simulink model "Hw1_4"  (R2015b)
settings: Solver=VariableStepAuto  StartTime=0.0  StopTime=5000  RelTol=1e-3
settings Model: Creator=user  LastModifiedBy=user

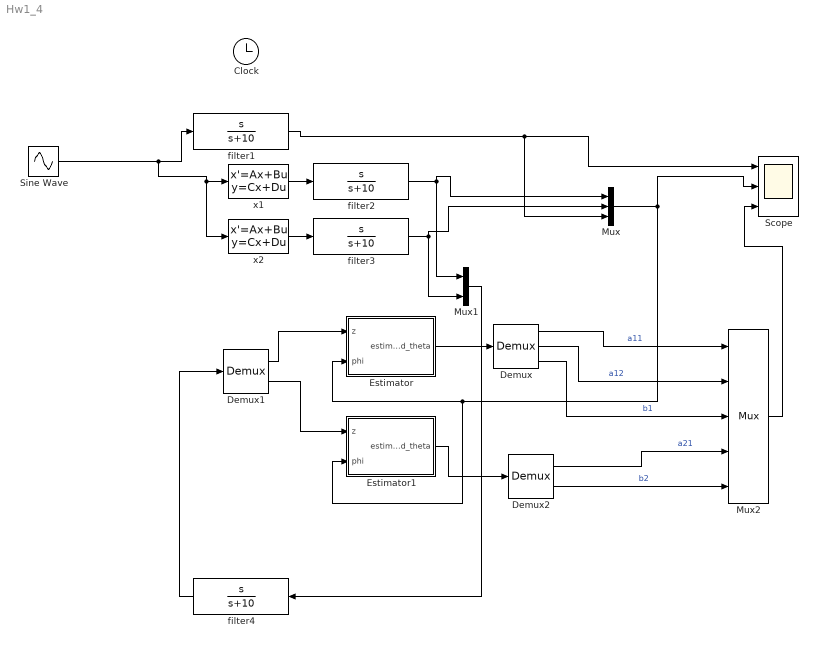
== system Hw1_4 ==
  Clock : Clock
      settings: Decimation=250
  Demux : Demux  Outputs=3
  Demux1 : Demux  Outputs=2
  Demux2 : Demux  Outputs=2
  Estimator : Subsystem
      mask Display: disp('Parameter\nEstimation')
  Estimator1 : Subsystem
      mask Display: disp('Parameter\nEstimation')
  Mux : Mux  Inputs=3
  Mux1 : Mux  Inputs=2
  Mux2 : Mux  Inputs=5
  Scope : Scope  NumInputPorts=3
  Sine Wave : Sin  Amplitude=10  Frequency=2  SampleTime=0
  filter{1..4} (4 alike) : TransferFcn  Numerator=[1 0]  Denominator=[1 10]
  x1 : StateSpace  A=[-0.25 3 ; -5 0 ]  B="[1  ; 2.2]"  C=[1 0]  D=0  X0=0
  x2 : StateSpace  A=[-0.25 3 ; -5 0 ]  B="[1  ; 2.2]"  C=[ 0 1]  D=0  X0=0
  wires:
  Sine Wave/1 -> x2/1, x1/1, filter1/1
  x1/1 -> filter2/1
  filter4/1 -> Demux1/1
  Estimator/1(estimated_theta) -> Demux/1
  x2/1 -> filter3/1
  Mux/1 -> Estimator1/2(phi), Estimator/2(phi), Scope/2
  Mux1/1 -> filter4/1
  Demux1/1 -> Estimator/1(z)
  Demux1/2 -> Estimator1/1(z)
  Estimator1/1(estimated_theta) -> Demux2/1
  Demux/1 -> Mux2/1  "a11"
  Demux/2 -> Mux2/2  "a12"
  Demux/3 -> Mux2/3  "b1"
  Demux2/1 -> Mux2/4  "a21"
  Demux2/2 -> Mux2/5  "b2"
  Mux2/1 -> Scope/3
  filter1/1 -> Mux/3, Scope/1
  filter2/1 -> Mux/1, Mux1/1
  filter3/1 -> Mux/2, Mux1/2

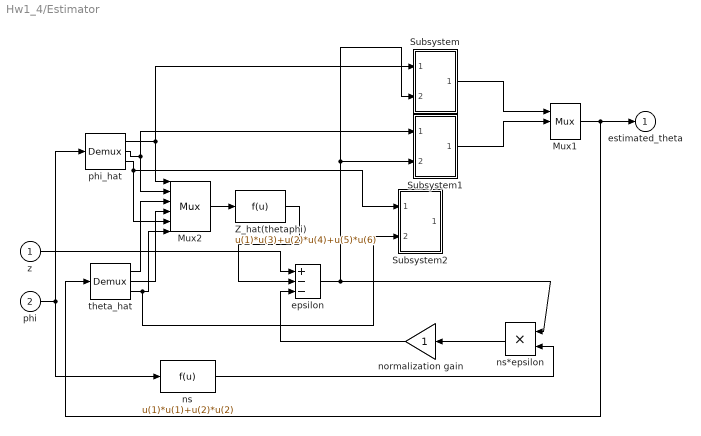
== system Hw1_4/Estimator ==
  z : Inport
  phi : Inport  Port=2
  Mux1 : Mux  Inputs=3
  Mux2 : Mux  Inputs=6
  Subsystem : Subsystem
  Subsystem1 : Subsystem
  Subsystem2 : Subsystem
  Z_hat(thetaphi) : Fcn  Expr=u(1)*u(3)+u(2)*u(4)+u(5)*u(6)
  epsilon : Sum  Inputs=+--  SaturateOnIntegerOverflow=on  InputSameDT=on  OutDataTypeStr=Inherit: Same as first input
  normalization gain : Gain  SaturateOnIntegerOverflow=on  OutDataTypeStr=Inherit: Same as input  ParamDataTypeStr=Inherit: Same as input
  ns : Fcn  Expr=u(1)*u(1)+u(2)*u(2)
      mask Display: disp('phi ''phi')
  ns*epsilon : Product  SaturateOnIntegerOverflow=on  RndMeth=Zero  InputSameDT=on  OutDataTypeStr=Inherit: Same as first input
  phi_hat : Demux  Outputs=3
  theta_hat : Demux  Outputs=3
  estimated_theta : Outport
  wires:
  z/1 -> epsilon/1
  normalization gain/1 -> epsilon/3
  phi_hat/1 -> Subsystem/1(In1), Mux2/1
  phi_hat/2 -> Mux2/2, Subsystem1/1(In1)
  Mux1/1 -> estimated_theta/1, theta_hat/1
  Z_hat(thetaphi)/1 -> epsilon/2
  phi/1 -> ns/1, phi_hat/1
  epsilon/1 -> ns*epsilon/1, Subsystem/2(In2), Subsystem1/2(In2)
  ns*epsilon/1 -> normalization gain/1
  theta_hat/1 -> Mux2/3
  theta_hat/2 -> Mux2/4
  Mux2/1 -> Z_hat(thetaphi)/1
  ns/1 -> ns*epsilon/2
  Subsystem/1(Out1) -> Mux1/1
  Subsystem1/1(Out1) -> Mux1/2
  phi_hat/3 -> Mux2/5, Subsystem2/1(In1)
  theta_hat/3 -> Subsystem2/2(In2), Mux2/6

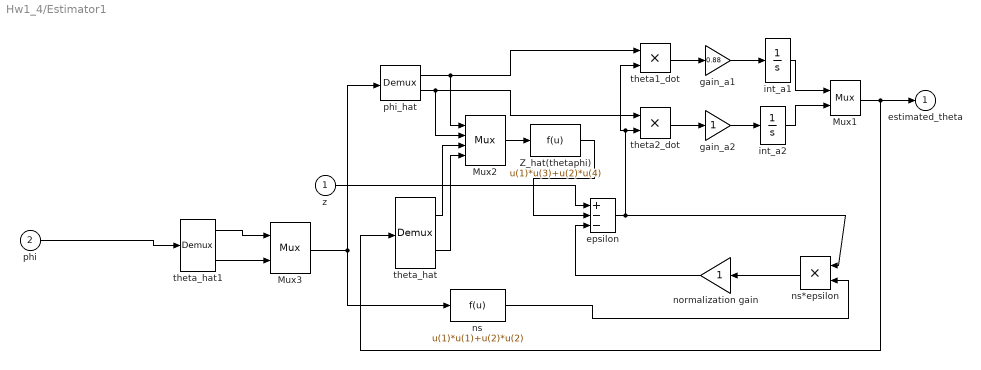
== system Hw1_4/Estimator1 ==
  z : Inport
  phi : Inport  Port=2
  Mux1 : Mux  Inputs=2
  Mux2 : Mux
  Mux3 : Mux  Inputs=2
  Z_hat(thetaphi) : Fcn  Expr=u(1)*u(3)+u(2)*u(4)
  epsilon : Sum  Inputs=+--  SaturateOnIntegerOverflow=on  InputSameDT=on  OutDataTypeStr=Inherit: Same as first input
  gain_a1 : Gain  Gain=0.88  SaturateOnIntegerOverflow=on  OutDataTypeStr=Inherit: Same as input  ParamDataTypeStr=Inherit: Same as input
  gain_a2 : Gain  SaturateOnIntegerOverflow=on  OutDataTypeStr=Inherit: Same as input  ParamDataTypeStr=Inherit: Same as input
  int_a1 : Integrator
  int_a2 : Integrator
  normalization gain : Gain  SaturateOnIntegerOverflow=on  OutDataTypeStr=Inherit: Same as input  ParamDataTypeStr=Inherit: Same as input
  ns : Fcn  Expr=u(1)*u(1)+u(2)*u(2)
      mask Display: disp('phi ''phi')
  ns*epsilon : Product  SaturateOnIntegerOverflow=on  RndMeth=Zero  InputSameDT=on  OutDataTypeStr=Inherit: Same as first input
  phi_hat : Demux  Outputs=2
  theta1_dot : Product  SaturateOnIntegerOverflow=on  RndMeth=Zero  InputSameDT=on  OutDataTypeStr=Inherit: Same as first input
  theta2_dot : Product  SaturateOnIntegerOverflow=on  RndMeth=Zero  InputSameDT=on  OutDataTypeStr=Inherit: Same as first input
  theta_hat : Demux  Outputs=2
  theta_hat1 : Demux  Outputs=3
  estimated_theta : Outport
  wires:
  z/1 -> epsilon/1
  normalization gain/1 -> epsilon/3
  phi_hat/1 -> theta1_dot/1, Mux2/1
  phi_hat/2 -> theta2_dot/1, Mux2/2
  Mux1/1 -> estimated_theta/1, theta_hat/1
  Z_hat(thetaphi)/1 -> epsilon/2
  phi/1 -> theta_hat1/1
  epsilon/1 -> ns*epsilon/1, theta1_dot/2, theta2_dot/2
  ns*epsilon/1 -> normalization gain/1
  int_a1/1 -> Mux1/1
  int_a2/1 -> Mux1/2
  theta_hat/1 -> Mux2/3
  theta_hat/2 -> Mux2/4
  Mux2/1 -> Z_hat(thetaphi)/1
  theta2_dot/1 -> gain_a2/1
  gain_a2/1 -> int_a2/1
  theta1_dot/1 -> gain_a1/1
  gain_a1/1 -> int_a1/1
  ns/1 -> ns*epsilon/2
  theta_hat1/3 -> Mux3/2
  theta_hat1/1 -> Mux3/1
  Mux3/1 -> ns/1, phi_hat/1

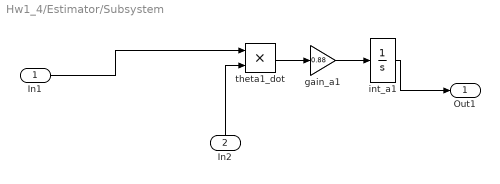
== system Hw1_4/Estimator/Subsystem ==
  In1 : Inport
  In2 : Inport  Port=2
  gain_a1 : Gain  Gain=0.88  SaturateOnIntegerOverflow=on  OutDataTypeStr=Inherit: Same as input  ParamDataTypeStr=Inherit: Same as input
  int_a1 : Integrator
  theta1_dot : Product  SaturateOnIntegerOverflow=on  RndMeth=Zero  InputSameDT=on  OutDataTypeStr=Inherit: Same as first input
  Out1 : Outport
  wires:
  theta1_dot/1 -> gain_a1/1
  gain_a1/1 -> int_a1/1
  int_a1/1 -> Out1/1
  In2/1 -> theta1_dot/2
  In1/1 -> theta1_dot/1

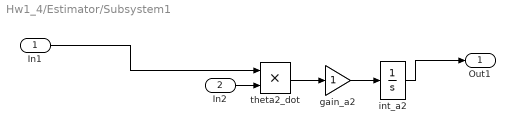
== system Hw1_4/Estimator/Subsystem1 ==
  In1 : Inport
  In2 : Inport  Port=2
  gain_a2 : Gain  SaturateOnIntegerOverflow=on  OutDataTypeStr=Inherit: Same as input  ParamDataTypeStr=Inherit: Same as input
  int_a2 : Integrator
  theta2_dot : Product  SaturateOnIntegerOverflow=on  RndMeth=Zero  InputSameDT=on  OutDataTypeStr=Inherit: Same as first input
  Out1 : Outport
  wires:
  int_a2/1 -> Out1/1
  theta2_dot/1 -> gain_a2/1
  gain_a2/1 -> int_a2/1
  In2/1 -> theta2_dot/2
  In1/1 -> theta2_dot/1

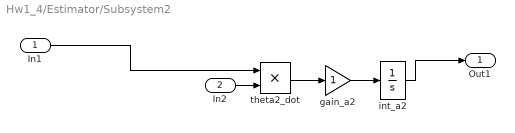
== system Hw1_4/Estimator/Subsystem2 ==
  In1 : Inport
  In2 : Inport  Port=2
  gain_a2 : Gain  SaturateOnIntegerOverflow=on  OutDataTypeStr=Inherit: Same as input  ParamDataTypeStr=Inherit: Same as input
  int_a2 : Integrator
  theta2_dot : Product  SaturateOnIntegerOverflow=on  RndMeth=Zero  InputSameDT=on  OutDataTypeStr=Inherit: Same as first input
  Out1 : Outport
  wires:
  int_a2/1 -> Out1/1
  theta2_dot/1 -> gain_a2/1
  gain_a2/1 -> int_a2/1
  In2/1 -> theta2_dot/2
  In1/1 -> theta2_dot/1
